simulink model "ControlManual"  (R2019a)
settings: Solver=VariableStepAuto  StartTime=0.0  StopTime=inf  RelTol=1e-3
settings Model: Creator=Usuario  LastModifiedBy=PATRICIA PEÑALOZA

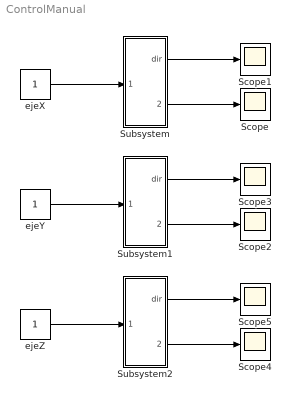
== system ControlManual ==
  Scope{,1..5} (6 alike) : Scope
  Subsystem : Subsystem
  Subsystem1 : Subsystem
  Subsystem2 : Subsystem
  ejeX : Constant
  ejeY : Constant
  ejeZ : Constant
  wires:
  ejeX/1 -> Subsystem/1(ejeX)
  Subsystem/1(dir) -> Scope1/1
  Subsystem/2(pul) -> Scope/1
  Subsystem1/2(pul) -> Scope2/1
  Subsystem1/1(dir) -> Scope3/1
  ejeY/1 -> Subsystem1/1(In1)
  ejeZ/1 -> Subsystem2/1(In1)
  Subsystem2/1(dir) -> Scope5/1
  Subsystem2/2(pul) -> Scope4/1

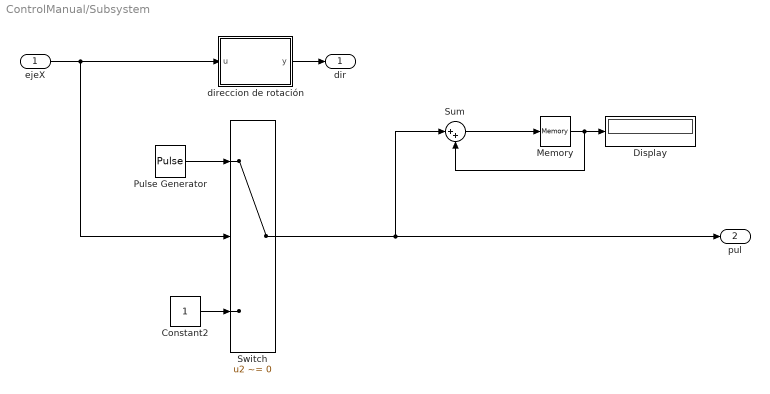
== system ControlManual/Subsystem ==
  ejeX : Inport
  Constant2 : Constant
  Display : Display
  Memory : Memory
  Pulse Generator : DiscretePulseGenerator  PulseType=Time based  PulseWidth=50  VectorParams1D=off
  Sum : Sum  Inputs=|++
  Switch : Switch  Criteria=u2 ~= 0
  direccion de rotación : MATLAB Function  TreatAsAtomicUnit=on
  dir : Outport
  pul : Outport  Port=2
  wires:
  direccion de rotación/1(y) -> dir/1
  Constant2/1 -> Switch/3
  Switch/1 -> Sum/1, pul/1
  Pulse Generator/1 -> Switch/1
  ejeX/1 -> Switch/2, direccion de rotación/1(u)
  Sum/1 -> Memory/1
  Memory/1 -> Sum/2, Display/1

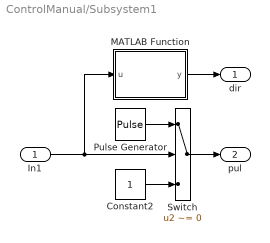
== system ControlManual/Subsystem1 ==
  In1 : Inport
  Constant2 : Constant
  MATLAB Function : MATLAB Function  TreatAsAtomicUnit=on
  Pulse Generator : DiscretePulseGenerator  PulseType=Time based  Period=0.5  PulseWidth=50
  Switch : Switch  Criteria=u2 ~= 0
  dir : Outport
  pul : Outport  Port=2
  wires:
  Pulse Generator/1 -> Switch/1
  Switch/1 -> pul/1
  Constant2/1 -> Switch/3
  In1/1 -> Switch/2, MATLAB Function/1(u)
  MATLAB Function/1(y) -> dir/1

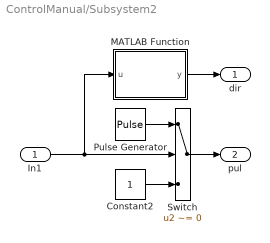
== system ControlManual/Subsystem2 ==
  In1 : Inport
  Constant2 : Constant
  MATLAB Function : MATLAB Function  TreatAsAtomicUnit=on
  Pulse Generator : DiscretePulseGenerator  PulseType=Time based  Period=0.5  PulseWidth=50
  Switch : Switch  Criteria=u2 ~= 0
  dir : Outport
  pul : Outport  Port=2
  wires:
  MATLAB Function/1(y) -> dir/1
  In1/1 -> MATLAB Function/1(u), Switch/2
  Constant2/1 -> Switch/3
  Switch/1 -> pul/1
  Pulse Generator/1 -> Switch/1

== matlab function ControlManual/Subsystem1/MATLAB Function ==
  data: u input; y output
function y = fcn(u)
if u>=0
    y=0;
else
    y=1;
end

== matlab function ControlManual/Subsystem/direccion de rotación ==
  data: u input; y output
function y = direction(u)
if u>=0
    y=0;
else
    y=1;
end

== matlab function ControlManual/Subsystem2/MATLAB Function ==
  data: u input; y output
function y = fcn(u)
if u>=0
    y=0;
else
    y=1;
end
